simulink model "NR_40MHz_3_1101"  (R2022b)
settings: Solver=VariableStepAuto  StartTime=0.0  StopTime=0.05  RelTol=1e-3
undefined symbols (not defined in the file): waveform
libraries: commutil2 x3, commrflib2 x1
(part 2 of 2)

== matlab function NR_40MHz_3_1101/5G NR Test Model ==
  data: wf output; waveform parameter; nsamps parameter; OutputAfterFinalValue parameter
function wf = wfGenerator(waveform, nsamps, OutputAfterFinalValue)

% Create persistent variable
persistent src;

% Preallocate output
wf = complex(zeros(nsamps,size(waveform,2)));

if isempty(src)
    % Get action when signal ends
    if OutputAfterFinalValue == 1
        signalEndAction = 'Cyclic repetition';
    else
        signalEndAction = 'Set to zero';
    end
    
    % Initialize persistent dsp.SignalSource to get current frame
    src = dsp.SignalSource(waveform,nsamps,'SignalEndAction',signalEndAction);
end

% Extract current frame
wf(:,:) = src();

end

== matlab function NR_40MHz_3_1101/5G NR Test Model2 ==
  data: wf output; waveform parameter; nsamps parameter; OutputAfterFinalValue parameter
function wf = wfGenerator(waveform, nsamps, OutputAfterFinalValue)

% Create persistent variable
persistent src;

% Preallocate output
wf = complex(zeros(nsamps,size(waveform,2)));

if isempty(src)
    % Get action when signal ends
    if OutputAfterFinalValue == 1
        signalEndAction = 'Cyclic repetition';
    else
        signalEndAction = 'Set to zero';
    end
    
    % Initialize persistent dsp.SignalSource to get current frame
    src = dsp.SignalSource(waveform,nsamps,'SignalEndAction',signalEndAction);
end

% Extract current frame
wf(:,:) = src();

end

== matlab function NR_40MHz_3_1101/5G NR Test Model3 ==
  data: wf output; waveform parameter; nsamps parameter; OutputAfterFinalValue parameter
function wf = wfGenerator(waveform, nsamps, OutputAfterFinalValue)

% Create persistent variable
persistent src;

% Preallocate output
wf = complex(zeros(nsamps,size(waveform,2)));

if isempty(src)
    % Get action when signal ends
    if OutputAfterFinalValue == 1
        signalEndAction = 'Cyclic repetition';
    else
        signalEndAction = 'Set to zero';
    end
    
    % Initialize persistent dsp.SignalSource to get current frame
    src = dsp.SignalSource(waveform,nsamps,'SignalEndAction',signalEndAction);
end

% Extract current frame
wf(:,:) = src();

end

== matlab function NR_40MHz_3_1101/5G NR Test Model5 ==
  data: wf output; waveform parameter; nsamps parameter; OutputAfterFinalValue parameter
function wf = wfGenerator(waveform, nsamps, OutputAfterFinalValue)

% Create persistent variable
persistent src;

% Preallocate output
wf = complex(zeros(nsamps,size(waveform,2)));

if isempty(src)
    % Get action when signal ends
    if OutputAfterFinalValue == 1
        signalEndAction = 'Cyclic repetition';
    else
        signalEndAction = 'Set to zero';
    end
    
    % Initialize persistent dsp.SignalSource to get current frame
    src = dsp.SignalSource(waveform,nsamps,'SignalEndAction',signalEndAction);
end

% Extract current frame
wf(:,:) = src();

end

== matlab function NR_40MHz_3_1101/5G NR Test Model7 ==
  data: wf output; waveform parameter; nsamps parameter; OutputAfterFinalValue parameter
function wf = wfGenerator(waveform, nsamps, OutputAfterFinalValue)

% Create persistent variable
persistent src;

% Preallocate output
wf = complex(zeros(nsamps,size(waveform,2)));

if isempty(src)
    % Get action when signal ends
    if OutputAfterFinalValue == 1
        signalEndAction = 'Cyclic repetition';
    else
        signalEndAction = 'Set to zero';
    end
    
    % Initialize persistent dsp.SignalSource to get current frame
    src = dsp.SignalSource(waveform,nsamps,'SignalEndAction',signalEndAction);
end

% Extract current frame
wf(:,:) = src();

end

== matlab function NR_40MHz_3_1101/5G NR Test Model1 ==
  data: wf output; waveform parameter; nsamps parameter; OutputAfterFinalValue parameter
function wf = wfGenerator(waveform, nsamps, OutputAfterFinalValue)

% Create persistent variable
persistent src;

% Preallocate output
wf = complex(zeros(nsamps,size(waveform,2)));

if isempty(src)
    % Get action when signal ends
    if OutputAfterFinalValue == 1
        signalEndAction = 'Cyclic repetition';
    else
        signalEndAction = 'Set to zero';
    end
    
    % Initialize persistent dsp.SignalSource to get current frame
    src = dsp.SignalSource(waveform,nsamps,'SignalEndAction',signalEndAction);
end

% Extract current frame
wf(:,:) = src();

end
